simulink model "FlSys_DetFlTnk"  (R2016b)
settings: configuration reference "CodeGenConfigSet" (kept outside this file)
values from neighbouring files (symbols this model uses):
  Fl_volTnkQnt_C = Calibration.Parameter    [init_FlSys_DetFlTnk.m]
  FlSys_dvolFlConsTnkLoMax_C = Calibration.Parameter    [init_FlSys_DetFlTnk.m]
  FlSys_dvolFlConsTnkLoMin_C = Calibration.Parameter    [init_FlSys_DetFlTnk.m]
  FlSys_swtTnkInfo_C = Calibration.Parameter    [init_FlSys_DetFlTnk.m]
  FlSys_volFlConsTnkHi_C = Calibration.Parameter    [init_FlSys_DetFlTnk.m]
  FlSys_volTnkHi_C = Calibration.Parameter    [init_FlSys_DetFlTnk.m]
  FlSys_volTnkLo_C = Calibration.Parameter    [init_FlSys_DetFlTnk.m]
undefined symbols (not defined in the file or in its folder): EngState_conv, SubSysExeState_conv, Switch_conv, SysExeState_conv
libraries: simulink x12, CXLib x4
settings Model: Creator=Administrator  LastModifiedBy=zhoutinglin
settings ConfigSetRef: SourceLocation=Base Workspace

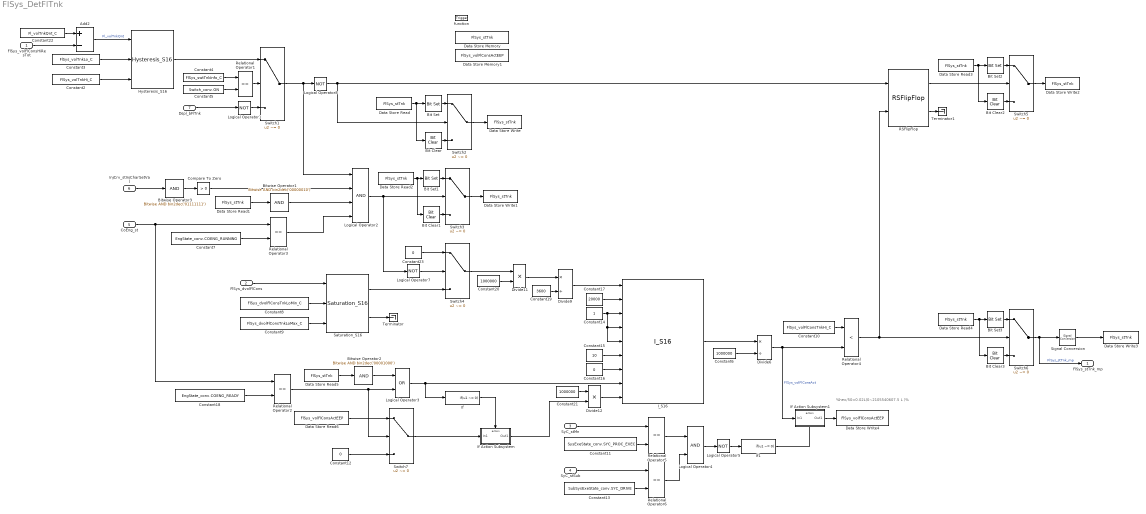
== system FlSys_DetFlTnk ==
  note: %hex/50=0.02L(0~2105540607.5 L )%
  FlSys_volFlConsHiResTot : Inport  Tag=L  Description=TotalFuelConsumption having higher resolution  OutMin=0  OutMax=4294967  OutDataTypeStr=FlConsum_L
  FlSys_dvolFlCons : Inport  Tag=L/h  Description=Fuel consumption [l/h]  Port=2  OutMin=0  OutMax=327  OutDataTypeStr=FlCon_L_h
  SyC_stMn : Inport  Description=Current system/ECU state  Port=3  OutDataTypeStr=Enum: SysExeState_conv
  SyC_stSub : Inport  Description=Current system/ECU sub-state  Port=4  OutDataTypeStr=Enum: SubSysExeState_conv
  CoEng_st : Inport  Description=Engine coordinator state  Port=5  OutDataTypeStr=Enum:EngState_conv
  InjCrv_stInjCharSetVal : Inport  Description=Injection characteristic setpoint (speed synchronous)  Port=6  OutMin=0  OutMax=255  OutDataTypeStr=State_uint8
  Dspl_bFlTnk : Inport  Description=Digital filling status of the fuel tank  Port=7  OutMin=0  OutMax=1  OutDataTypeStr=boolean
  function : TriggerPort  TriggerType=function-call  VariantControl=Variant
  Add2 : Sum  Inputs=+-  OutDataTypeStr=Inherit: Inherit via back propagation  SaturateOnIntegerOverflow=on  InputSameDT=on
  Bit Clear : simulink/Logic and Bit Operations/Bit Clear  iBit=0
  Bit Clear1 : simulink/Logic and Bit Operations/Bit Clear  iBit=2
  Bit Clear2 : simulink/Logic and Bit Operations/Bit Clear  iBit=1
  Bit Clear3 : simulink/Logic and Bit Operations/Bit Clear  iBit=3
  Bit Set : simulink/Logic and Bit Operations/Bit Set  iBit=0
  Bit Set1 : simulink/Logic and Bit Operations/Bit Set  iBit=2
  Bit Set2 : simulink/Logic and Bit Operations/Bit Set  iBit=1
  Bit Set3 : simulink/Logic and Bit Operations/Bit Set  iBit=3
  Bitwise Operator1 : simulink/Logic and Bit Operations/Bitwise Operator  logicop=AND  UseBitMask=on  BitMask=bin2dec('00000010')  BitMaskRealWorld=Stored Integer
  Bitwise Operator2 : simulink/Logic and Bit Operations/Bitwise Operator  logicop=AND  UseBitMask=on  BitMask=bin2dec('00001000')  BitMaskRealWorld=Stored Integer
  Bitwise Operator3 : simulink/Logic and Bit Operations/Bitwise Operator  logicop=AND  UseBitMask=on  BitMask=bin2dec('01111111')  BitMaskRealWorld=Stored Integer
  Compare To Zero : simulink/Logic and Bit Operations/Compare To Zero  relop=>  OutDataTypeStr=boolean
  Constant10 : Constant  Value=FlSys_volFlConsTnkHi_C
  Constant11 : Constant  Value=SysExeState_conv.SYC_PROC_EXEC
  Constant12 : Constant  Value=0  OutDataTypeStr=Inherit: Inherit via back propagation
  Constant13 : Constant  Value=SubSysExeState_conv.SYC_DRIVE
  Constant14 : Constant  OutDataTypeStr=Inherit: Inherit via back propagation
  Constant15 : Constant  Value=10  OutDataTypeStr=Inherit: Inherit via back propagation
  Constant16 : Constant  Value=0  OutDataTypeStr=Inherit: Inherit via back propagation
  Constant17 : Constant  Value=20000  OutDataTypeStr=uint32
  Constant18 : Constant  Value=EngState_conv.COENG_READY
  Constant19 : Constant  Value=3600  OutDataTypeStr=uint16
  Constant2 : Constant  Value=FlSys_volTnkHi_C
  Constant20 : Constant  Value=1000000  OutDataTypeStr=int32
  Constant21 : Constant  Value=1000000  OutDataTypeStr=int32
  Constant22 : Constant  Value=Fl_volTnkQnt_C
  Constant23 : Constant  Value=0  OutDataTypeStr=Inherit: Inherit via back propagation
  Constant3 : Constant  Value=FlSys_volTnkLo_C
  Constant4 : Constant  Value=FlSys_swtTnkInfo_C
  Constant5 : Constant  Value=Switch_conv.ON
  Constant6 : Constant  Value=1000000  OutDataTypeStr=int32
  Constant7 : Constant  Value=EngState_conv.COENG_RUNNING
  Constant8 : Constant  Value=FlSys_dvolFlConsTnkLoMin_C
  Constant9 : Constant  Value=FlSys_dvolFlConsTnkLoMax_C
  Data Store Memory : DataStoreMemory  DataStoreName=FlSys_stTnk  ReadBeforeWriteMsg=warning  WriteAfterWriteMsg=warning  WriteAfterReadMsg=warning  ShowAdditionalParam=off  StateMustResolveToSignalObject=on
  Data Store Memory1 : DataStoreMemory  DataStoreName=FlSys_volFlConsActEEP  ReadBeforeWriteMsg=warning  WriteAfterWriteMsg=warning  WriteAfterReadMsg=warning  ShowAdditionalParam=off
  Data Store Read{,1..5} (6 alike) : DataStoreRead  DataStoreName=FlSys_stTnk
  Data Store Read6 : DataStoreRead  DataStoreName=FlSys_volFlConsActEEP
  Data Store Write{,1..3} (4 alike) : DataStoreWrite  DataStoreName=FlSys_stTnk
  Data Store Write4 : DataStoreWrite  DataStoreName=FlSys_volFlConsActEEP
  Divide11 : Product  Inputs=**  OutDataTypeStr=int32  SaturateOnIntegerOverflow=on
  Divide12 : Product  Inputs=**  OutDataTypeStr=uint32  SaturateOnIntegerOverflow=on
  Divide6 : Product  Inputs=*/  OutDataTypeStr=Inherit: Inherit via back propagation  SaturateOnIntegerOverflow=on
  Divide9 : Product  Inputs=*/  OutDataTypeStr=int32  SaturateOnIntegerOverflow=on
  Hysteresis_S16 : CXLib/Hysteresis_S16
  I_S16 : CXLib/I_S16
  If : If  IfExpression=u1 ~= 0  ShowElse=off
  If Action Subsystem : Subsystem  TreatAsAtomicUnit=on
  If Action Subsystem1 : Subsystem  TreatAsAtomicUnit=on
  If1 : If  IfExpression=u1 ~= 0  ShowElse=off
  Logical Operator{1,5,7..8} (4 alike) : Logic  Operator=NOT  AllPortsSameDT=off  OutDataTypeStr=boolean
  Logical Operator2 : Logic  Inputs=4  AllPortsSameDT=off  OutDataTypeStr=boolean
  Logical Operator3 : Logic  Operator=OR  AllPortsSameDT=off  OutDataTypeStr=boolean
  Logical Operator4 : Logic  AllPortsSameDT=off  OutDataTypeStr=boolean
  RSFlipFlop : CXLib/RSFlipFlop
  Relational Operator{1..3,5..6} (5 alike) : RelationalOperator  Operator===  OutDataTypeStr=boolean  RndMeth=Simplest  InputSameDT=on
  Relational Operator4 : RelationalOperator  Operator=<  OutDataTypeStr=boolean  RndMeth=Simplest  InputSameDT=on
  Saturation_S16 : CXLib/Saturation_S16
  Signal Conversion : SignalConversion  OverrideOpt=off
  Switch{1..7} (7 alike) : Switch  Criteria=u2 ~= 0  SaturateOnIntegerOverflow=on  InputSameDT=on
  Terminator : Terminator
  Terminator1 : Terminator
  FlSys_stTnk_mp : Outport  Description=bit-coded message for tank level  OutMin=0  OutMax=255  OutDataTypeStr=State_uint8
  wires:
  FlSys_volFlConsHiResTot/1 -> Add2/2
  Constant3/1 -> Hysteresis_S16/2
  Constant2/1 -> Hysteresis_S16/3
  Dspl_bFlTnk/1 -> Logical Operator1/1
  Logical Operator1/1 -> Switch1/3
  Constant4/1 -> Relational Operator1/1
  Constant5/1 -> Relational Operator1/2
  Relational Operator1/1 -> Switch1/2
  InjCrv_stInjCharSetVal/1 -> Bitwise Operator3/1
  Switch1/1 -> Logical Operator2/1, Logical Operator8/1
  Compare To Zero/1 -> Logical Operator2/2
  Bit Clear/1 -> Switch2/3
  Bit Set/1 -> Switch2/1
  Data Store Read/1 -> Bit Clear/1, Bit Set/1
  Switch2/1 -> Data Store Write/1
  Bitwise Operator1/1 -> Logical Operator2/3
  Data Store Read1/1 -> Bitwise Operator1/1
  CoEng_st/1 -> Relational Operator2/1, Relational Operator3/1
  Constant7/1 -> Relational Operator3/2
  Relational Operator3/1 -> Logical Operator2/4
  Logical Operator2/1 -> Switch3/2, Logical Operator7/1
  Bit Clear1/1 -> Switch3/3
  Bit Set1/1 -> Switch3/1
  Data Store Read2/1 -> Bit Set1/1, Bit Clear1/1
  Switch3/1 -> Data Store Write1/1
  Saturation_S16/2 -> Terminator/1
  FlSys_dvolFlCons/1 -> Saturation_S16/1
  Constant8/1 -> Saturation_S16/2
  Constant9/1 -> Saturation_S16/3
  Saturation_S16/1 -> Switch4/3
  Constant23/1 -> Switch4/1
  Divide9/1 -> I_S16/1
  Divide6/1 -> Relational Operator4/2, If Action Subsystem1/1(In1)  "FlSys_volFlConsAct"
  Constant10/1 -> Relational Operator4/1
  RSFlipFlop/2 -> Terminator1/1
  RSFlipFlop/1 -> Switch5/2
  Bit Clear2/1 -> Switch5/3
  Bit Set2/1 -> Switch5/1
  Data Store Read3/1 -> Bit Set2/1, Bit Clear2/1
  Switch5/1 -> Data Store Write2/1
  Relational Operator4/1 -> RSFlipFlop/2, Switch6/2
  Bit Clear3/1 -> Switch6/3
  Bit Set3/1 -> Switch6/1
  Data Store Read4/1 -> Bit Clear3/1, Bit Set3/1
  Bitwise Operator2/1 -> Logical Operator3/1
  Data Store Read5/1 -> Bitwise Operator2/1
  Relational Operator2/1 -> Switch7/2, Logical Operator3/2
  Logical Operator3/1 -> I_S16/8, If/1
  If/1 -> If Action Subsystem/Action
  Switch7/1 -> If Action Subsystem/1(In1)
  Constant12/1 -> Switch7/3
  Data Store Read6/1 -> Switch7/1
  If Action Subsystem/1(Out1) -> Divide12/2
  SyC_stMn/1 -> Relational Operator5/1
  Constant11/1 -> Relational Operator5/2
  Constant13/1 -> Relational Operator6/2
  SyC_stSub/1 -> Relational Operator6/1
  Relational Operator5/1 -> Logical Operator4/1
  Relational Operator6/1 -> Logical Operator4/2
  Logical Operator4/1 -> Logical Operator5/1
  If Action Subsystem1/1(Out1) -> Data Store Write4/1
  If1/1 -> If Action Subsystem1/Action
  Constant14/1 -> I_S16/5, I_S16/4, I_S16/3
  Constant15/1 -> I_S16/6
  Constant16/1 -> I_S16/7
  Constant17/1 -> I_S16/2
  Logical Operator5/1 -> If1/1
  Bitwise Operator3/1 -> Compare To Zero/1
  Switch6/1 -> FlSys_stTnk_mp/1, Signal Conversion/1  "FlSys_stTnk_mp"
  Constant6/1 -> Divide6/2
  I_S16/1 -> Divide6/1
  Hysteresis_S16/1 -> Switch1/1
  Constant18/1 -> Relational Operator2/2
  Constant19/1 -> Divide9/2
  Constant20/1 -> Divide11/2
  Divide11/1 -> Divide9/1
  Switch4/1 -> Divide11/1
  Constant21/1 -> Divide12/1
  Divide12/1 -> I_S16/9
  Constant22/1 -> Add2/1
  Add2/1 -> Hysteresis_S16/1  "Fl_volTnkQnt"
  Logical Operator7/1 -> Switch4/2
  Logical Operator8/1 -> RSFlipFlop/1, Switch2/2
  Signal Conversion/1 -> Data Store Write3/1

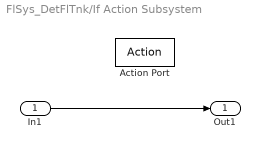
== system FlSys_DetFlTnk/If Action Subsystem ==
  In1 : Inport
  Action Port : ActionPort  ActionType=then
  Out1 : Outport
  wires:
  In1/1 -> Out1/1

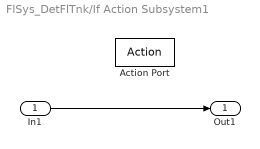
== system FlSys_DetFlTnk/If Action Subsystem1 ==
  In1 : Inport
  Action Port : ActionPort  ActionType=then
  Out1 : Outport
  wires:
  In1/1 -> Out1/1
